simulink model "ZZC_quadrotor_20251110_v3"  (R2019b)
settings: Solver=ode4  StartTime=0.0  StopTime=100  FixedStep=1e-3
libraries: simulink x5
settings Model: Creator=bitgar  LastModifiedBy=bitgar

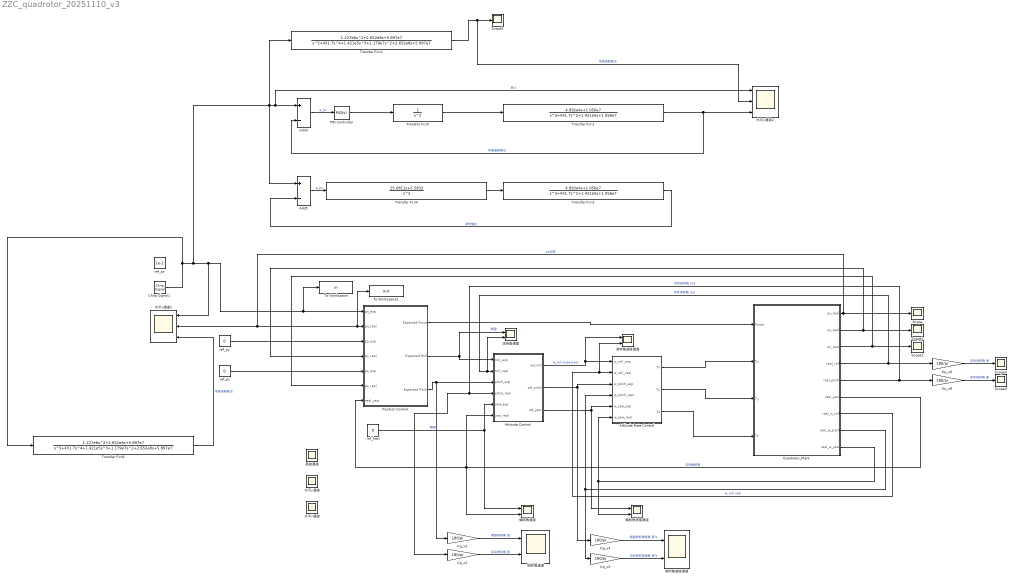
== system ZZC_quadrotor_20251110_v3 ==
  Add3 : Sum  Inputs=+-
  Add5 : Sum  Inputs=+-
  Attitude Control : Subsystem
  Attitude Rate Control : Subsystem
  Chirp Signal1 : simulink/Sources/Chirp Signal  f1=0.0001  T=100  f2=100
  Kp_x{2..6,8} (6 alike) : Gain  Gain=180/pi
  PID Controller : simulink/Continuous/PID Controller  Controller=PID  Form=Parallel  TimeDomain=Continuous-time  SampleTime=-1  IntegratorMethod=Forward Euler  FilterMethod=Forward Euler  ControllerParametersSource=internal  P=5.5832  I=0  D=25.0811  UseFilter=on  N=1000  TunerSelectOption=Transfer Function Based (PID Tuner App)  InitialConditionSource=internal  InitialConditionForIntegrator=0  InitialConditionForFilter=0  DifferentiatorICPrevScaledInput=0  ExternalReset=none  TrackingMode=off  Kt=1  LimitOutput=off  UpperSaturationLimit=inf  LowerSaturationLimit=-inf  LinearizeAsGain=on  AntiWindupMode=none  Kb=1  POutMin=[]  POutMax=[]  IOutMin=[]  IOutMax=[]  DOutMin=[]  DOutMax=[]  NOutMin=[]  NOutMax=[]  SumOutMin=[]  SumOutMax=[]  SaturationOutMin=[]  SaturationOutMax=[]  PParamMin=[]  PParamMax=[]  IParamMin=[]  IParamMax=[]  DParamMin=[]  DParamMax=[]  NParamMin=[]  NParamMax=[]  KbParamMin=[]  KbParamMax=[]  KtParamMin=[]  KtParamMax=[]  KbOutMin=[]  KbOutMax=[]  KtOutMin=[]  KtOutMax=[]  IntegratorOutMin=[]  IntegratorOutMax=[]  FilterOutMin=[]  FilterOutMax=[]  SumI1OutMin=[]  SumI1OutMax=[]  SumI2OutMin=[]  SumI2OutMax=[]  SumI3OutMin=[]  SumI3OutMax=[]  SumI4OutMin=[]  SumI4OutMax=[]  SumDOutMin=[]  SumDOutMax=[]  DifferentiatorOutMin=[]  DifferentiatorOutMax=[]  FilterDiffOutCoefMin=[]  FilterDiffOutCoefMax=[]  ReciprocalOutMin=[]  ReciprocalOutMax=[]  SumDenOutMin=[]  SumDenOutMax=[]  SumNumOutMin=[]  SumNumOutMax=[]  DivideOutMin=[]  DivideOutMax=[]  IntegratorContinuousStateAttributes=''  IntegratorStateMustResolveToSignalObject=off  IntegratorRTWStateStorageClass=Auto  FilterContinuousStateAttributes=''  FilterStateMustResolveToSignalObject=off  FilterRTWStateStorageClass=Auto  ParallelPVariant=InternalParameters  IdealPVariant=Disabled  IVariant=InternalParameters  DVariant=InternalParameters  IntegratorVariant=Continuous  SatVariant=Disabled  AWVariant=Passthrough  PCopyVariant=Disabled  TRVariant=Disabled  FdbkBlocksVariant=Forward  IdealPFdbkVariant=Disabled  SatFdbkVariant=Disabled  DerivativeFilterVariant=ContFilter  NVariant=InternalParameters  NCopyVariant=Disabled  FilterICVariant=InternalICsFilter  IntegratorICVariant=InternalICs  ExternalResetVariant=Disabled  TRSumVariant=Passthrough  SumFdbkVariant=Disabled  SumVariant=Sum_PID
  Position Control : Subsystem
  Quadrotor_Plant : Subsystem
  Scope{,1..5} (6 alike) : Scope
  To Workspace : ToWorkspace  VariableName=in  SampleTime=-1
  To Workspace1 : ToWorkspace  VariableName=out  SampleTime=-1
  Transfer Fcn1 : TransferFcn  Numerator=[4.892e4 1.056e7]  Denominator=[1 431.7 1.421e5 1.056e7]
  Transfer Fcn2 : TransferFcn  Numerator=[1.227e6 2.652e8 5.897e7]  Denominator=[1 431.7 1.421e5 1.179e7 2.652e8 5.897e7]
  Transfer Fcn3 : TransferFcn  Numerator=[4.892e4 1.056e7]  Denominator=[1 431.7 1.421e5 1.056e7]
  Transfer Fcn4 : TransferFcn  Numerator=[0 25.0811 5.5832]  Denominator=[1 0 0]
  Transfer Fcn5 : TransferFcn  Denominator=[1 0 0]
  Transfer Fcn8 : TransferFcn  Numerator=[1.227e6 2.652e8 5.897e7]  Denominator=[1 431.7 1.421e5 1.179e7 2.652e8 5.897e7]
  ref_kesi : Constant  Value=0
  ref_px : Constant  Value=1e-2
  ref_py : Constant  Value=0
  ref_pz : Constant  Value=0
  俯仰角通道 : Scope  NumInputPorts=2
  俯仰角速度通道 : Scope  NumInputPorts=2
  偏航角通道 : Scope  NumInputPorts=2
  偏航角速度通道 : Scope  NumInputPorts=2
  水平x通道 : Scope  NumInputPorts=2
  水平x通道1 : Scope  NumInputPorts=3
  水平x通道2 : Scope  NumInputPorts=3
  水平y通道 : Scope  NumInputPorts=2
  滚转角通道 : Scope  NumInputPorts=2
  滚转角速度通道 : Scope  NumInputPorts=2
  高度通道 : Scope  NumInputPorts=2
  wires:
  Quadrotor_Plant/4(real_roll) -> Kp_x6/1, 滚转角通道/2, Attitude Control/2(roll_real)  "实际滚转角 rad"
  Attitude Control/2(wd_pitch) -> Attitude Rate Control/3(w_pitch_exp), Kp_x4/1
  Attitude Control/1(wd_roll) -> 滚转角速度通道/1, Attitude Rate Control/1(w_roll_exp)  "w_roll expected"
  ref_py/1 -> Position Control/3(py_exp)
  Position Control/1(Expected Force) -> Quadrotor_Plant/1(Force)
  ref_pz/1 -> Position Control/5(pz_exp)
  ref_kesi/1 -> Attitude Control/5(yaw_exp), 偏航角通道/1  "期望"
  Quadrotor_Plant/2(py_real) -> Position Control/4(py_real), Scope1/1
  Quadrotor_Plant/1(px_real) -> 水平x通道1/2, To Workspace1/1, Position Control/2(px_real), Scope/1  "px反馈"
  Attitude Rate Control/1(Tx) -> Quadrotor_Plant/2(Tx)
  Attitude Rate Control/2(Ty) -> Quadrotor_Plant/3(Ty)
  Attitude Rate Control/3(Tz) -> Quadrotor_Plant/4(Tz)
  Quadrotor_Plant/7(real_w_roll) -> 滚转角速度通道/2, Attitude Rate Control/2(w_roll_real)  "w_roll real"
  Quadrotor_Plant/8(real_w_pitch) -> Kp_x5/1, Attitude Rate Control/4(w_pitch_real)
  Quadrotor_Plant/9(real_w_yaw) -> 偏航角速度通道/2, Attitude Rate Control/6(w_yaw_real)
  Attitude Control/3(wd_yaw) -> Attitude Rate Control/5(w_yaw_exp), 偏航角速度通道/1
  Position Control/2(Expected Roll) -> 滚转角通道/1, Attitude Control/1(roll_exp)  "期望"
  Position Control/3(Expected Pitch) -> Attitude Control/3(pitch_exp), Kp_x3/1
  Transfer Fcn2/1 -> 水平x通道2/2, Scope5/1  "传递函数输出"
  Kp_x2/1 -> 俯仰角通道/2  "实际俯仰角 度"
  Kp_x3/1 -> 俯仰角通道/1  "期望俯仰角 度"
  Kp_x4/1 -> 俯仰角速度通道/1  "期望俯仰角速度 度/s"
  Kp_x5/1 -> 俯仰角速度通道/2  "实际俯仰角速度 度/s"
  Quadrotor_Plant/5(real_pitch) -> Kp_x8/1, Kp_x2/1, Attitude Control/4(pitch_real)  "实际俯仰角 rad"
  Quadrotor_Plant/6(real_yaw) -> 偏航角通道/2, Position Control/7(real_yaw), Attitude Control/6(yaw_real)  "实际偏航角"
  Quadrotor_Plant/3(pz_real) -> Scope2/1, Position Control/6(pz_real)
  Kp_x6/1 -> Scope3/1  "实际滚转角 度"
  Kp_x8/1 -> Scope4/1  "实际俯仰角 度"
  Chirp Signal1/1 -> Transfer Fcn8/1, Transfer Fcn2/1, Add5/1, 水平x通道2/1, Add3/1, 水平x通道1/1, To Workspace/1, Position Control/1(px_exp)  "输入"
  Transfer Fcn1/1 -> 水平x通道2/3, Add3/2  "传递函数输出"
  Transfer Fcn4/1 -> Transfer Fcn3/1
  Add5/1 -> Transfer Fcn4/1  "e_px"
  Transfer Fcn3/1 -> Add5/2  "新的输出"
  Add3/1 -> PID Controller/1  "e_px"
  Transfer Fcn8/1 -> 水平x通道1/3  "传递函数输出"
  PID Controller/1 -> Transfer Fcn5/1
  Transfer Fcn5/1 -> Transfer Fcn1/1

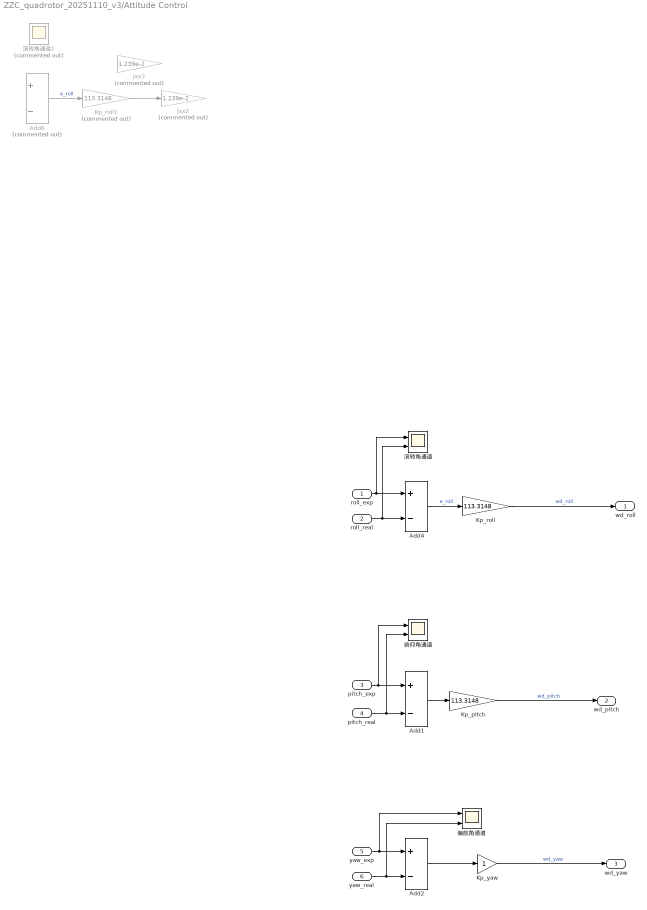
== system ZZC_quadrotor_20251110_v3/Attitude Control ==
  roll_exp : Inport
  roll_real : Inport  Port=2
  pitch_exp : Inport  Port=3
  pitch_real : Inport  Port=4
  yaw_exp : Inport  Port=5
  yaw_real : Inport  Port=6
  Add1 : Sum  Inputs=+-
  Add2 : Sum  Inputs=+-
  Add4 : Sum  Inputs=+-
  Add6 : Sum  Commented=on  Inputs=+-
  Jxx2 : Gain  Commented=on  Gain=1.239e-2
  Jxx3 : Gain  Commented=on  Gain=1.239e-2
  Kp_pitch : Gain  Gain=113.3148
  Kp_roll : Gain  Gain=113.3148
  Kp_roll1 : Gain  Commented=on  Gain=113.3148
  Kp_yaw : Gain
  俯仰角通道 : Scope  NumInputPorts=2
  偏航角通道 : Scope  NumInputPorts=2
  滚转角通道 : Scope  NumInputPorts=2
  滚转角通道1 : Scope  Commented=on  NumInputPorts=2
  wd_roll : Outport
  wd_pitch : Outport  Port=2
  wd_yaw : Outport  Port=3
  wires:
  roll_exp/1 -> 滚转角通道/1, Add4/1
  roll_real/1 -> 滚转角通道/2, Add4/2
  pitch_exp/1 -> 俯仰角通道/1, Add1/1
  pitch_real/1 -> 俯仰角通道/2, Add1/2
  yaw_real/1 -> 偏航角通道/2, Add2/2
  Add4/1 -> Kp_roll/1  "e_roll"
  yaw_exp/1 -> 偏航角通道/1, Add2/1
  Add1/1 -> Kp_pitch/1
  Add2/1 -> Kp_yaw/1
  Kp_roll/1 -> wd_roll/1  "wd_roll"
  Kp_pitch/1 -> wd_pitch/1  "wd_pitch"
  Kp_yaw/1 -> wd_yaw/1  "wd_yaw"
  Add6/1 -> Kp_roll1/1  "e_roll"
  Kp_roll1/1 -> Jxx2/1

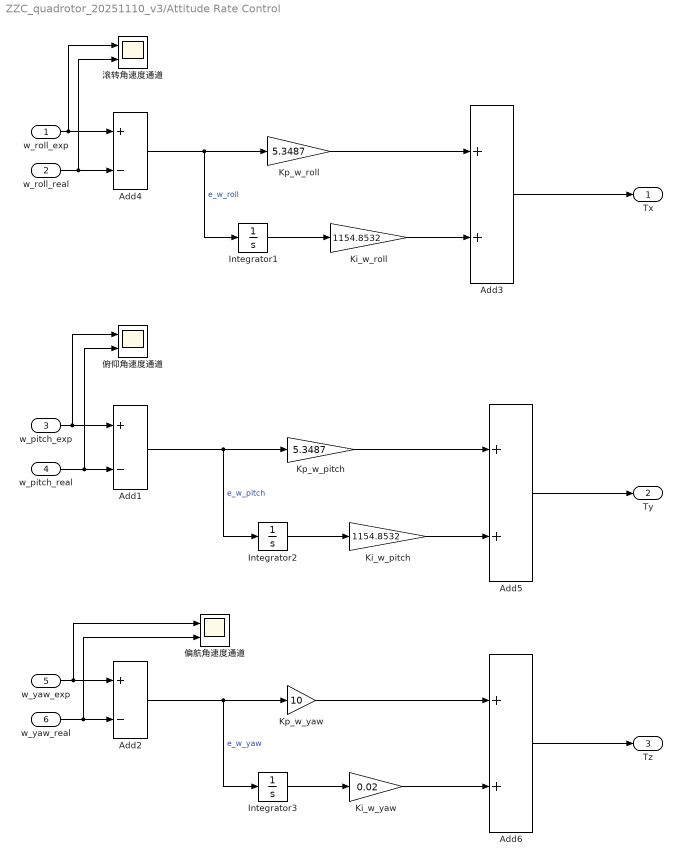
== system ZZC_quadrotor_20251110_v3/Attitude Rate Control ==
  w_roll_exp : Inport
  w_roll_real : Inport  Port=2
  w_pitch_exp : Inport  Port=3
  w_pitch_real : Inport  Port=4
  w_yaw_exp : Inport  Port=5
  w_yaw_real : Inport  Port=6
  Add1 : Sum  Inputs=+-
  Add2 : Sum  Inputs=+-
  Add3 : Sum
  Add4 : Sum  Inputs=+-
  Add5 : Sum
  Add6 : Sum
  Integrator1 : Integrator
  Integrator2 : Integrator
  Integrator3 : Integrator
  Ki_w_pitch : Gain  Gain=1154.8532
  Ki_w_roll : Gain  Gain=1154.8532
  Ki_w_yaw : Gain  Gain=0.02
  Kp_w_pitch : Gain  Gain=5.3487
  Kp_w_roll : Gain  Gain=5.3487
  Kp_w_yaw : Gain  Gain=10
  俯仰角速度通道 : Scope  NumInputPorts=2
  偏航角速度通道 : Scope  NumInputPorts=2
  滚转角速度通道 : Scope  NumInputPorts=2
  Tx : Outport
  Ty : Outport  Port=2
  Tz : Outport  Port=3
  wires:
  w_roll_exp/1 -> 滚转角速度通道/1, Add4/1
  w_roll_real/1 -> 滚转角速度通道/2, Add4/2
  w_pitch_exp/1 -> 俯仰角速度通道/1, Add1/1
  w_pitch_real/1 -> 俯仰角速度通道/2, Add1/2
  w_yaw_real/1 -> 偏航角速度通道/2, Add2/2
  Add4/1 -> Integrator1/1, Kp_w_roll/1  "e_w_roll"
  w_yaw_exp/1 -> 偏航角速度通道/1, Add2/1
  Add3/1 -> Tx/1
  Ki_w_roll/1 -> Add3/2
  Kp_w_roll/1 -> Add3/1
  Integrator1/1 -> Ki_w_roll/1
  Integrator2/1 -> Ki_w_pitch/1
  Kp_w_pitch/1 -> Add5/1
  Ki_w_pitch/1 -> Add5/2
  Add1/1 -> Integrator2/1, Kp_w_pitch/1  "e_w_pitch"
  Add5/1 -> Ty/1
  Add2/1 -> Integrator3/1, Kp_w_yaw/1  "e_w_yaw"
  Integrator3/1 -> Ki_w_yaw/1
  Kp_w_yaw/1 -> Add6/1
  Ki_w_yaw/1 -> Add6/2
  Add6/1 -> Tz/1

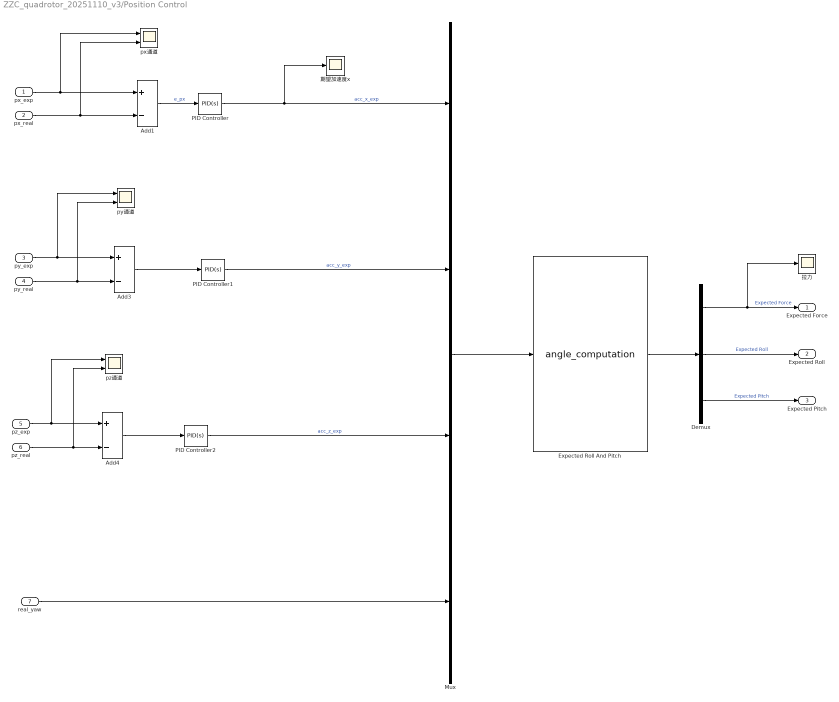
== system ZZC_quadrotor_20251110_v3/Position Control ==
  px_exp : Inport
  px_real : Inport  Port=2
  py_exp : Inport  Port=3
  py_real : Inport  Port=4
  pz_exp : Inport  Port=5
  pz_real : Inport  Port=6
  real_yaw : Inport  Port=7
  Add1 : Sum  Inputs=+-
  Add3 : Sum  Inputs=+-
  Add4 : Sum  Inputs=+-
  Demux : Demux  Outputs=3
  Expected Roll And Pitch : S-Function  FunctionName=angle_computation  Parameters=1 9.81  SFunctionDeploymentMode=off  EnableBusSupport=off
  Mux : Mux
  PID Controller : simulink/Continuous/PID Controller  Controller=PID  Form=Parallel  TimeDomain=Continuous-time  SampleTime=-1  IntegratorMethod=Forward Euler  FilterMethod=Forward Euler  ControllerParametersSource=internal  P=5.5832  I=0  D=25.0811  UseFilter=on  N=1000  TunerSelectOption=Transfer Function Based (PID Tuner App)  InitialConditionSource=internal  InitialConditionForIntegrator=0  InitialConditionForFilter=0  DifferentiatorICPrevScaledInput=0  ExternalReset=none  TrackingMode=off  Kt=1  LimitOutput=off  UpperSaturationLimit=inf  LowerSaturationLimit=-inf  LinearizeAsGain=on  AntiWindupMode=none  Kb=1  POutMin=[]  POutMax=[]  IOutMin=[]  IOutMax=[]  DOutMin=[]  DOutMax=[]  NOutMin=[]  NOutMax=[]  SumOutMin=[]  SumOutMax=[]  SaturationOutMin=[]  SaturationOutMax=[]  PParamMin=[]  PParamMax=[]  IParamMin=[]  IParamMax=[]  DParamMin=[]  DParamMax=[]  NParamMin=[]  NParamMax=[]  KbParamMin=[]  KbParamMax=[]  KtParamMin=[]  KtParamMax=[]  KbOutMin=[]  KbOutMax=[]  KtOutMin=[]  KtOutMax=[]  IntegratorOutMin=[]  IntegratorOutMax=[]  FilterOutMin=[]  FilterOutMax=[]  SumI1OutMin=[]  SumI1OutMax=[]  SumI2OutMin=[]  SumI2OutMax=[]  SumI3OutMin=[]  SumI3OutMax=[]  SumI4OutMin=[]  SumI4OutMax=[]  SumDOutMin=[]  SumDOutMax=[]  DifferentiatorOutMin=[]  DifferentiatorOutMax=[]  FilterDiffOutCoefMin=[]  FilterDiffOutCoefMax=[]  ReciprocalOutMin=[]  ReciprocalOutMax=[]  SumDenOutMin=[]  SumDenOutMax=[]  SumNumOutMin=[]  SumNumOutMax=[]  DivideOutMin=[]  DivideOutMax=[]  IntegratorContinuousStateAttributes=''  IntegratorStateMustResolveToSignalObject=off  IntegratorRTWStateStorageClass=Auto  FilterContinuousStateAttributes=''  FilterStateMustResolveToSignalObject=off  FilterRTWStateStorageClass=Auto  ParallelPVariant=InternalParameters  IdealPVariant=Disabled  IVariant=InternalParameters  DVariant=InternalParameters  IntegratorVariant=Continuous  SatVariant=Disabled  AWVariant=Passthrough  PCopyVariant=Disabled  TRVariant=Disabled  FdbkBlocksVariant=Forward  IdealPFdbkVariant=Disabled  SatFdbkVariant=Disabled  DerivativeFilterVariant=ContFilter  NVariant=InternalParameters  NCopyVariant=Disabled  FilterICVariant=InternalICsFilter  IntegratorICVariant=InternalICs  ExternalResetVariant=Disabled  TRSumVariant=Passthrough  SumFdbkVariant=Disabled  SumVariant=Sum_PID
  PID Controller1 : simulink/Continuous/PID Controller  Controller=PID  Form=Parallel  TimeDomain=Continuous-time  SampleTime=-1  IntegratorMethod=Forward Euler  FilterMethod=Forward Euler  ControllerParametersSource=internal  P=5.5832  I=0  D=25.0811  UseFilter=on  N=1000  TunerSelectOption=Transfer Function Based (PID Tuner App)  InitialConditionSource=internal  InitialConditionForIntegrator=0  InitialConditionForFilter=0  DifferentiatorICPrevScaledInput=0  ExternalReset=none  TrackingMode=off  Kt=1  LimitOutput=off  UpperSaturationLimit=inf  LowerSaturationLimit=-inf  LinearizeAsGain=on  AntiWindupMode=none  Kb=1  POutMin=[]  POutMax=[]  IOutMin=[]  IOutMax=[]  DOutMin=[]  DOutMax=[]  NOutMin=[]  NOutMax=[]  SumOutMin=[]  SumOutMax=[]  SaturationOutMin=[]  SaturationOutMax=[]  PParamMin=[]  PParamMax=[]  IParamMin=[]  IParamMax=[]  DParamMin=[]  DParamMax=[]  NParamMin=[]  NParamMax=[]  KbParamMin=[]  KbParamMax=[]  KtParamMin=[]  KtParamMax=[]  KbOutMin=[]  KbOutMax=[]  KtOutMin=[]  KtOutMax=[]  IntegratorOutMin=[]  IntegratorOutMax=[]  FilterOutMin=[]  FilterOutMax=[]  SumI1OutMin=[]  SumI1OutMax=[]  SumI2OutMin=[]  SumI2OutMax=[]  SumI3OutMin=[]  SumI3OutMax=[]  SumI4OutMin=[]  SumI4OutMax=[]  SumDOutMin=[]  SumDOutMax=[]  DifferentiatorOutMin=[]  DifferentiatorOutMax=[]  FilterDiffOutCoefMin=[]  FilterDiffOutCoefMax=[]  ReciprocalOutMin=[]  ReciprocalOutMax=[]  SumDenOutMin=[]  SumDenOutMax=[]  SumNumOutMin=[]  SumNumOutMax=[]  DivideOutMin=[]  DivideOutMax=[]  IntegratorContinuousStateAttributes=''  IntegratorStateMustResolveToSignalObject=off  IntegratorRTWStateStorageClass=Auto  FilterContinuousStateAttributes=''  FilterStateMustResolveToSignalObject=off  FilterRTWStateStorageClass=Auto  ParallelPVariant=InternalParameters  IdealPVariant=Disabled  IVariant=InternalParameters  DVariant=InternalParameters  IntegratorVariant=Continuous  SatVariant=Disabled  AWVariant=Passthrough  PCopyVariant=Disabled  TRVariant=Disabled  FdbkBlocksVariant=Forward  IdealPFdbkVariant=Disabled  SatFdbkVariant=Disabled  DerivativeFilterVariant=ContFilter  NVariant=InternalParameters  NCopyVariant=Disabled  FilterICVariant=InternalICsFilter  IntegratorICVariant=InternalICs  ExternalResetVariant=Disabled  TRSumVariant=Passthrough  SumFdbkVariant=Disabled  SumVariant=Sum_PID
  PID Controller2 : simulink/Continuous/PID Controller  Controller=PID  Form=Parallel  TimeDomain=Continuous-time  SampleTime=-1  IntegratorMethod=Forward Euler  FilterMethod=Forward Euler  ControllerParametersSource=internal  P=10  I=0  D=2  UseFilter=on  N=1000  TunerSelectOption=Transfer Function Based (PID Tuner App)  InitialConditionSource=internal  InitialConditionForIntegrator=0  InitialConditionForFilter=0  DifferentiatorICPrevScaledInput=0  ExternalReset=none  TrackingMode=off  Kt=1  LimitOutput=off  UpperSaturationLimit=inf  LowerSaturationLimit=-inf  LinearizeAsGain=on  AntiWindupMode=none  Kb=1  POutMin=[]  POutMax=[]  IOutMin=[]  IOutMax=[]  DOutMin=[]  DOutMax=[]  NOutMin=[]  NOutMax=[]  SumOutMin=[]  SumOutMax=[]  SaturationOutMin=[]  SaturationOutMax=[]  PParamMin=[]  PParamMax=[]  IParamMin=[]  IParamMax=[]  DParamMin=[]  DParamMax=[]  NParamMin=[]  NParamMax=[]  KbParamMin=[]  KbParamMax=[]  KtParamMin=[]  KtParamMax=[]  KbOutMin=[]  KbOutMax=[]  KtOutMin=[]  KtOutMax=[]  IntegratorOutMin=[]  IntegratorOutMax=[]  FilterOutMin=[]  FilterOutMax=[]  SumI1OutMin=[]  SumI1OutMax=[]  SumI2OutMin=[]  SumI2OutMax=[]  SumI3OutMin=[]  SumI3OutMax=[]  SumI4OutMin=[]  SumI4OutMax=[]  SumDOutMin=[]  SumDOutMax=[]  DifferentiatorOutMin=[]  DifferentiatorOutMax=[]  FilterDiffOutCoefMin=[]  FilterDiffOutCoefMax=[]  ReciprocalOutMin=[]  ReciprocalOutMax=[]  SumDenOutMin=[]  SumDenOutMax=[]  SumNumOutMin=[]  SumNumOutMax=[]  DivideOutMin=[]  DivideOutMax=[]  IntegratorContinuousStateAttributes=''  IntegratorStateMustResolveToSignalObject=off  IntegratorRTWStateStorageClass=Auto  FilterContinuousStateAttributes=''  FilterStateMustResolveToSignalObject=off  FilterRTWStateStorageClass=Auto  ParallelPVariant=InternalParameters  IdealPVariant=Disabled  IVariant=InternalParameters  DVariant=InternalParameters  IntegratorVariant=Continuous  SatVariant=Disabled  AWVariant=Passthrough  PCopyVariant=Disabled  TRVariant=Disabled  FdbkBlocksVariant=Forward  IdealPFdbkVariant=Disabled  SatFdbkVariant=Disabled  DerivativeFilterVariant=ContFilter  NVariant=InternalParameters  NCopyVariant=Disabled  FilterICVariant=InternalICsFilter  IntegratorICVariant=InternalICs  ExternalResetVariant=Disabled  TRSumVariant=Passthrough  SumFdbkVariant=Disabled  SumVariant=Sum_PID
  px通道 : Scope  NumInputPorts=2
  py通道 : Scope  NumInputPorts=2
  pz通道 : Scope  NumInputPorts=2
  拉力 : Scope
  期望加速度x : Scope
  Expected Force : Outport
  Expected Roll : Outport  Port=2
  Expected Pitch : Outport  Port=3
  wires:
  Add1/1 -> PID Controller/1  "e_px"
  Mux/1 -> Expected Roll And Pitch/1
  Expected Roll And Pitch/1 -> Demux/1
  Demux/2 -> Expected Roll/1  "Expected Roll"
  Demux/3 -> Expected Pitch/1  "Expected Pitch"
  px_exp/1 -> Add1/1, px通道/1
  px_real/1 -> Add1/2, px通道/2
  Add3/1 -> PID Controller1/1
  py_exp/1 -> Add3/1, py通道/1
  py_real/1 -> Add3/2, py通道/2
  pz_exp/1 -> pz通道/1, Add4/1
  pz_real/1 -> Add4/2, pz通道/2
  Demux/1 -> 拉力/1, Expected Force/1  "Expected Force"
  PID Controller2/1 -> Mux/3  "acc_z_exp"
  PID Controller1/1 -> Mux/2  "acc_y_exp"
  PID Controller/1 -> 期望加速度x/1, Mux/1  "acc_x_exp"
  real_yaw/1 -> Mux/4
  Add4/1 -> PID Controller2/1

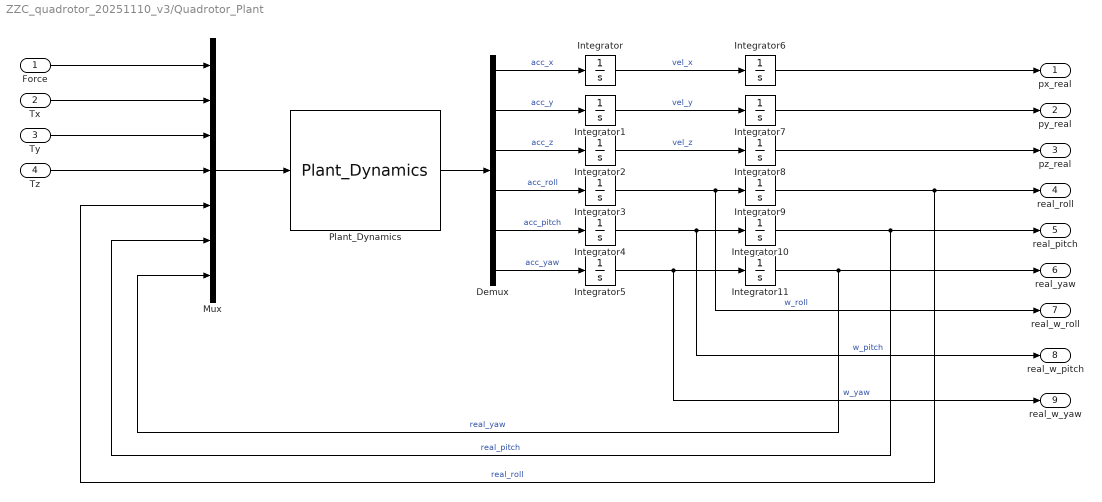
== system ZZC_quadrotor_20251110_v3/Quadrotor_Plant ==
  Force : Inport
  Tx : Inport  Port=2
  Ty : Inport  Port=3
  Tz : Inport  Port=4
  Demux : Demux  Outputs=6
  Integrator{,1..11} (12 alike) : Integrator
  Mux : Mux  Inputs=7
  Plant_Dynamics : S-Function  FunctionName=Plant_Dynamics  Parameters=1 9.81 0.01239 0.01239 0.02382  SFunctionDeploymentMode=off  EnableBusSupport=off
  px_real : Outport
  py_real : Outport  Port=2
  pz_real : Outport  Port=3
  real_roll : Outport  Port=4
  real_pitch : Outport  Port=5
  real_yaw : Outport  Port=6
  real_w_roll : Outport  Port=7
  real_w_pitch : Outport  Port=8
  real_w_yaw : Outport  Port=9
  wires:
  Demux/4 -> Integrator3/1  "acc_roll"
  Integrator6/1 -> px_real/1
  Mux/1 -> Plant_Dynamics/1
  Demux/3 -> Integrator2/1  "acc_z"
  Integrator/1 -> Integrator6/1  "vel_x"
  Tx/1 -> Mux/2
  Integrator1/1 -> Integrator7/1  "vel_y"
  Demux/1 -> Integrator/1  "acc_x"
  Integrator8/1 -> pz_real/1
  Demux/5 -> Integrator4/1  "acc_pitch"
  Demux/6 -> Integrator5/1  "acc_yaw"
  Integrator2/1 -> Integrator8/1  "vel_z"
  Demux/2 -> Integrator1/1  "acc_y"
  Tz/1 -> Mux/4
  Integrator7/1 -> py_real/1
  Force/1 -> Mux/1
  Ty/1 -> Mux/3
  Integrator9/1 -> real_roll/1, Mux/5  "real_roll"
  Integrator10/1 -> real_pitch/1, Mux/6  "real_pitch"
  Plant_Dynamics/1 -> Demux/1
  Integrator11/1 -> real_yaw/1, Mux/7  "real_yaw"
  Integrator3/1 -> real_w_roll/1, Integrator9/1  "w_roll"
  Integrator4/1 -> real_w_pitch/1, Integrator10/1  "w_pitch"
  Integrator5/1 -> real_w_yaw/1, Integrator11/1  "w_yaw"
